simulink model "generic_20231123_1032"  (R2022b)
settings: Solver=ode45  StartTime=0.0  StopTime=50  RelTol=1e-3  EnableMultiTasking=on
model workspace (MAT data in the model file):
  A = 1
  Amplifier = -9.10007585438
  B = 1.19071237887
  K_d_yawrate = 0.231634180251
  K_dsteering = 5.24463953925
  k_speed = -0.570636497542
  k_stanley = 28.4909595466
  kd = -9.99955278144
  ki = 0.00519416981022
  kp = 9.99999979837
  path_curvature = 0
values from neighbouring files (symbols this model uses):
  brake_select = ones(length(speed), length(steering_angle))    [TwoDLook_uptable.m]
  curvature = 0.000:0.001:1    [TwoDLook_uptable.m]
  m = 1600    [MPCController1.m]    (also in MPCController2.m; MPC_Fmincon.m)
  speed = 0:0.1:100    [TwoDLook_uptable.m]
  steering_angle = -3.14/4:0.00628/4:3.14/4    [TwoDLook_uptable.m]
undefined symbols (not defined in the file or in its folder): DiscIntNeverNeededParam
libraries: CarMaker4SL x143, simulink x11, cstblocks x6, simulink_extras x4, autolibshared x1, mpcadaslib x1
(part 3 of 7)

== system generic_20231123_1032/CarMaker/IPG Vehicle/CarAndTrailer/Forces/Vehicle Forces ==
  Sync_In : Inport
  Bus Creator1 : BusCreator  Inputs=12
  Bus Creator8 : BusCreator  Inputs=16
  BusCreator1 : BusCreator  Inputs=4
  BusCreator2 : BusCreator  Inputs=9
  Demux : Demux  Outputs=16
      settings: DisplayOption=none
  Demux1 : Demux  Outputs=12
      settings: DisplayOption=none
  Demux2 : Demux  Outputs=13
      settings: DisplayOption=none
  Forces : S-Function  FunctionName=CM_Sfun  Parameters='Forces'  SFunctionDeploymentMode=off  EnableBusSupport=off
  Terminator : Terminator
  Sync_Out : Outport  VectorParamsAs1DForOutWhenUnconnected=off
  Car.Virtual : Outport  Port=2  VectorParamsAs1DForOutWhenUnconnected=off
  Car.Aero : Outport  Port=3  VectorParamsAs1DForOutWhenUnconnected=off
  Car.Load : Outport  Port=4  VectorParamsAs1DForOutWhenUnconnected=off
  wires:
  BusCreator1/1 -> Terminator/1  "Aero IF (in)"
  Demux2/13 -> BusCreator2/9  "car Aero Trq_1 z"
  Demux2/12 -> BusCreator2/8  "car Aero Trq_1 y"
  Demux2/11 -> BusCreator2/7  "car Aero Trq_1 x"
  Demux2/10 -> BusCreator2/6  "car Aero Frc_1 z"
  Demux2/9 -> BusCreator2/5  "car Aero Frc_1 y"
  Demux2/8 -> BusCreator2/4  "car Aero Frc_1 x"
  Demux2/7 -> BusCreator2/3  "car Aero PoA_1 z"
  Demux2/6 -> BusCreator2/2  "car Aero PoA_1 y"
  Demux2/5 -> BusCreator2/1  "car Aero PoA_1 x"
  Demux2/4 -> BusCreator1/4  "car Aero tau_1"
  Demux2/3 -> BusCreator1/3  "car Aero ApproachVel_1 z"
  Demux2/2 -> BusCreator1/2  "car Aero ApproachVel_1 y"
  Demux2/1 -> BusCreator1/1  "car Aero ApproachVel_1 x"
  Demux/16 -> Bus Creator8/16  "Car Load_3 tz"
  Demux/15 -> Bus Creator8/15  "Car Load_3 ty"
  Demux/14 -> Bus Creator8/14  "Car Load_3 tx"
  Demux/13 -> Bus Creator8/13  "Car Load_3 mass"
  Demux1/12 -> Bus Creator1/12  "Car Virtual Trq_0 z"
  Demux1/11 -> Bus Creator1/11  "Car Virtual Trq_0 y"
  Demux1/10 -> Bus Creator1/10  "Car Virtual Trq_0 x"
  Demux1/9 -> Bus Creator1/9  "Car Virtual Trq_1 z"
  Demux1/8 -> Bus Creator1/8  "Car Virtual Trq_1 y"
  Demux1/7 -> Bus Creator1/7  "Car Virtual Trq_1 x"
  Demux1/6 -> Bus Creator1/6  "Car Virtual Frc_0 z"
  Demux1/5 -> Bus Creator1/5  "Car Virtual Frc_0 y"
  Demux1/4 -> Bus Creator1/4  "Car Virtual Frc_0 x"
  Sync_In/1 -> Forces/1
  Forces/1 -> Sync_Out/1
  BusCreator2/1 -> Car.Aero/1
  Demux1/1 -> Bus Creator1/1  "Car Virtual Frc_1 x"
  Demux1/2 -> Bus Creator1/2  "Car Virtual Frc_1 y"
  Demux1/3 -> Bus Creator1/3  "Car Virtual Frc_1 z"
  Forces/3 -> Demux2/1
  Forces/2 -> Demux1/1
  Bus Creator1/1 -> Car.Virtual/1
  Bus Creator8/1 -> Car.Load/1
  Demux/1 -> Bus Creator8/1  "Car Load_0 mass"
  Demux/2 -> Bus Creator8/2  "Car Load_0 tx"
  Demux/3 -> Bus Creator8/3  "Car Load_0 ty"
  Demux/4 -> Bus Creator8/4  "Car Load_0 tz"
  Demux/5 -> Bus Creator8/5  "Car Load_1 mass"
  Demux/6 -> Bus Creator8/6  "Car Load_1 tx"
  Demux/7 -> Bus Creator8/7  "Car Load_1 ty"
  Demux/8 -> Bus Creator8/8  "Car Load_1 tz"
  Demux/9 -> Bus Creator8/9  "Car Load_2 mass"
  Demux/10 -> Bus Creator8/10  "Car Load_2 tx"
  Demux/11 -> Bus Creator8/11  "Car Load_2 ty"
  Demux/12 -> Bus Creator8/12  "Car Load_2 tz"
  Forces/4 -> Demux/1

== system generic_20231123_1032/CarMaker/IPG Vehicle/CarAndTrailer/Trailer/CreateBus Car.Hitch.FrcTrq ==
  In1 : Inport
  Bus Creator7 : BusCreator  Inputs=6
  Demux7 : Demux  Outputs=6
      settings: DisplayOption=none
  Out1 : Outport  VectorParamsAs1DForOutWhenUnconnected=off
  wires:
  In1/1 -> Demux7/1
  Bus Creator7/1 -> Out1/1
  Demux7/6 -> Bus Creator7/6  "Car Hitch Trq2Car z"
  Demux7/5 -> Bus Creator7/5  "Car Hitch Trq2Car y"
  Demux7/4 -> Bus Creator7/4  "Car Hitch Trq2Car x"
  Demux7/3 -> Bus Creator7/3  "Car Hitch Frc2Car z"
  Demux7/2 -> Bus Creator7/2  "Car Hitch Frc2Car y"
  Demux7/1 -> Bus Creator7/1  "Car Hitch Frc2Car x"

== system generic_20231123_1032/CarMaker/IPG Vehicle/CarAndTrailer/Trailer/CreateBus Vhcl.Motion ==
  In1 : Inport
  BusCreator : BusCreator  Inputs=15
  Demux : Demux  Outputs=15
      settings: DisplayOption=none
  Out1 : Outport  VectorParamsAs1DForOutWhenUnconnected=off
  wires:
  Demux/15 -> BusCreator/15  "Vhcl YawAcc"
  Demux/14 -> BusCreator/14  "Vhcl YawVel"
  Demux/13 -> BusCreator/13  "Vhcl Yaw"
  Demux/12 -> BusCreator/12  "Vhcl PitchAcc"
  Demux/11 -> BusCreator/11  "Vhcl PitchVel"
  Demux/10 -> BusCreator/10  "Vhcl Pitch"
  Demux/9 -> BusCreator/9  "Vhcl RollAcc"
  Demux/8 -> BusCreator/8  "Vhcl RollVel"
  Demux/7 -> BusCreator/7  "Vhcl Roll"
  Demux/6 -> BusCreator/6  "Vhcl Hitch_Pos z"
  Demux/5 -> BusCreator/5  "Vhcl Hitch_Pos y"
  Demux/4 -> BusCreator/4  "Vhcl Hitch_Pos x"
  Demux/3 -> BusCreator/3  "Vhcl sRoad"
  Demux/2 -> BusCreator/2  "Vhcl Distance"
  Demux/1 -> BusCreator/1  "Vhcl v"
  In1/1 -> Demux/1
  BusCreator/1 -> Out1/1

== system generic_20231123_1032/CarMaker/IPG Vehicle/CarAndTrailer/Trailer/CreateBus Vhcl.PoI ==
  In1 : Inport
  Bus Creator3 : BusCreator  Inputs=18
  Demux3 : Demux  Outputs=18
      settings: DisplayOption=none
  Out1 : Outport  VectorParamsAs1DForOutWhenUnconnected=off
  wires:
  Demux3/18 -> Bus Creator3/18  "Vhcl PoI_GCS Elev"
  Demux3/17 -> Bus Creator3/17  "Vhcl PoI_GCS Lat"
  Demux3/16 -> Bus Creator3/16  "Vhcl PoI_GCS Long"
  Demux3/15 -> Bus Creator3/15  "Vhcl PoI_Acc_1 z"
  Demux3/14 -> Bus Creator3/14  "Vhcl PoI_Acc_1 y"
  Demux3/13 -> Bus Creator3/13  "Vhcl PoI_Acc_1 x"
  Demux3/12 -> Bus Creator3/12  "Vhcl PoI_Vel_1 z"
  Demux3/11 -> Bus Creator3/11  "Vhcl PoI_Vel_1 y"
  Demux3/10 -> Bus Creator3/10  "Vhcl PoI_Vel_1 x"
  Demux3/9 -> Bus Creator3/9  "Vhcl PoI_Acc z"
  Demux3/8 -> Bus Creator3/8  "Vhcl PoI_Acc y"
  Demux3/7 -> Bus Creator3/7  "Vhcl PoI_Acc x"
  Demux3/6 -> Bus Creator3/6  "Vhcl PoI_Vel z"
  Demux3/5 -> Bus Creator3/5  "Vhcl PoI_Vel y"
  Demux3/4 -> Bus Creator3/4  "Vhcl PoI_Vel x"
  Demux3/3 -> Bus Creator3/3  "Vhcl PoI_Pos z"
  Demux3/2 -> Bus Creator3/2  "Vhcl PoI_Pos y"
  In1/1 -> Demux3/1
  Bus Creator3/1 -> Out1/1
  Demux3/1 -> Bus Creator3/1  "Vhcl PoI_Pos x"

== system generic_20231123_1032/CarMaker/IPG Vehicle/CarAndTrailer/Trailer/CreateBus Vhcl.Steering ==
  In1 : Inport
  Bus Creator3 : BusCreator  Inputs=4
  Demux : Demux
      settings: DisplayOption=none
  Out1 : Outport  VectorParamsAs1DForOutWhenUnconnected=off
  wires:
  Bus Creator3/1 -> Out1/1
  Demux/1 -> Bus Creator3/1  "Vhcl Steering Ang"
  Demux/3 -> Bus Creator3/3  "Vhcl Steering AngAcc"
  Demux/2 -> Bus Creator3/2  "Vhcl Steering AngVel"
  Demux/4 -> Bus Creator3/4  "Vhcl Steering Trq"
  In1/1 -> Demux/1

== system generic_20231123_1032/CarMaker/IPG Vehicle/CarAndTrailer/Trailer/CreateBus Vhcl.Wheel.FL ==
  In1 : Inport
  Bus Creator3 : BusCreator  Inputs=14
  Demux3 : Demux  Outputs=14
      settings: DisplayOption=none
  Out1 : Outport  VectorParamsAs1DForOutWhenUnconnected=off
  wires:
  Demux3/14 -> Bus Creator3/14  "Vhcl Wheel FL Trq_WhlBearing"
  Demux3/13 -> Bus Creator3/13  "Vhcl Wheel FL Trq_T2W"
  Demux3/12 -> Bus Creator3/12  "Vhcl Wheel FL SideSlip"
  Demux3/11 -> Bus Creator3/11  "Vhcl Wheel FL LongSlip"
  Demux3/10 -> Bus Creator3/10  "Vhcl Wheel FL vBelt"
  Demux3/9 -> Bus Creator3/9  "Vhcl Wheel FL Fz"
  Demux3/8 -> Bus Creator3/8  "Vhcl Wheel FL Fy"
  Demux3/7 -> Bus Creator3/7  "Vhcl Wheel FL Fx"
  Demux3/6 -> Bus Creator3/6  "Vhcl Wheel FL r_zxy z"
  Demux3/5 -> Bus Creator3/5  "Vhcl Wheel FL r_zxy y"
  Demux3/4 -> Bus Creator3/4  "Vhcl Wheel FL r_zxy x"
  Demux3/3 -> Bus Creator3/3  "Vhcl Wheel FL t z"
  Demux3/2 -> Bus Creator3/2  "Vhcl Wheel FL t y"
  In1/1 -> Demux3/1
  Bus Creator3/1 -> Out1/1
  Demux3/1 -> Bus Creator3/1  "Vhcl Wheel FL t x"

== system generic_20231123_1032/CarMaker/IPG Vehicle/CarAndTrailer/Trailer/CreateBus Vhcl.Wheel.FR ==
  In1 : Inport
  Bus Creator3 : BusCreator  Inputs=14
  Demux3 : Demux  Outputs=14
      settings: DisplayOption=none
  Out1 : Outport  VectorParamsAs1DForOutWhenUnconnected=off
  wires:
  Demux3/14 -> Bus Creator3/14  "Vhcl Wheel FR Trq_WhlBearing"
  Demux3/13 -> Bus Creator3/13  "Vhcl Wheel FR Trq_T2W"
  Demux3/12 -> Bus Creator3/12  "Vhcl Wheel FR SideSlip"
  Demux3/11 -> Bus Creator3/11  "Vhcl Wheel FR LongSlip"
  Demux3/10 -> Bus Creator3/10  "Vhcl Wheel FR vBelt"
  Demux3/9 -> Bus Creator3/9  "Vhcl Wheel FR Fz"
  Demux3/8 -> Bus Creator3/8  "Vhcl Wheel FR Fy"
  Demux3/7 -> Bus Creator3/7  "Vhcl Wheel FR Fx"
  Demux3/6 -> Bus Creator3/6  "Vhcl Wheel FR r_zxy z"
  Demux3/5 -> Bus Creator3/5  "Vhcl Wheel FR r_zxy y"
  Demux3/4 -> Bus Creator3/4  "Vhcl Wheel FR r_zxy x"
  Demux3/3 -> Bus Creator3/3  "Vhcl Wheel FR t z"
  Demux3/2 -> Bus Creator3/2  "Vhcl Wheel FR t y"
  In1/1 -> Demux3/1
  Bus Creator3/1 -> Out1/1
  Demux3/1 -> Bus Creator3/1  "Vhcl Wheel FR t x"

== system generic_20231123_1032/CarMaker/IPG Vehicle/CarAndTrailer/Trailer/CreateBus Vhcl.Wheel.RL ==
  In1 : Inport
  Bus Creator3 : BusCreator  Inputs=14
  Demux3 : Demux  Outputs=14
      settings: DisplayOption=none
  Out1 : Outport  VectorParamsAs1DForOutWhenUnconnected=off
  wires:
  Demux3/14 -> Bus Creator3/14  "Vhcl Wheel RL Trq_WhlBearing"
  Demux3/13 -> Bus Creator3/13  "Vhcl Wheel RL Trq_T2W"
  Demux3/12 -> Bus Creator3/12  "Vhcl Wheel RL SideSlip"
  Demux3/11 -> Bus Creator3/11  "Vhcl Wheel RL LongSlip"
  Demux3/10 -> Bus Creator3/10  "Vhcl Wheel RL vBelt"
  Demux3/9 -> Bus Creator3/9  "Vhcl Wheel RL Fz"
  Demux3/8 -> Bus Creator3/8  "Vhcl Wheel RL Fy"
  Demux3/7 -> Bus Creator3/7  "Vhcl Wheel RL Fx"
  Demux3/6 -> Bus Creator3/6  "Vhcl Wheel RL r_zxy z"
  Demux3/5 -> Bus Creator3/5  "Vhcl Wheel RL r_zxy y"
  Demux3/4 -> Bus Creator3/4  "Vhcl Wheel RL r_zxy x"
  Demux3/3 -> Bus Creator3/3  "Vhcl Wheel RL t z"
  Demux3/2 -> Bus Creator3/2  "Vhcl Wheel RL t y"
  In1/1 -> Demux3/1
  Bus Creator3/1 -> Out1/1
  Demux3/1 -> Bus Creator3/1  "Vhcl Wheel RL t x"

== system generic_20231123_1032/CarMaker/IPG Vehicle/CarAndTrailer/Trailer/CreateBus Vhcl.Wheel.RR ==
  In1 : Inport
  Bus Creator3 : BusCreator  Inputs=14
  Demux3 : Demux  Outputs=14
      settings: DisplayOption=none
  Out1 : Outport  VectorParamsAs1DForOutWhenUnconnected=off
  wires:
  Demux3/14 -> Bus Creator3/14  "Vhcl Wheel RR Trq_WhlBearing"
  Demux3/13 -> Bus Creator3/13  "Vhcl Wheel RR Trq_T2W"
  Demux3/12 -> Bus Creator3/12  "Vhcl Wheel RR SideSlip"
  Demux3/11 -> Bus Creator3/11  "Vhcl Wheel RR LongSlip"
  Demux3/10 -> Bus Creator3/10  "Vhcl Wheel RR vBelt"
  Demux3/9 -> Bus Creator3/9  "Vhcl Wheel RR Fz"
  Demux3/8 -> Bus Creator3/8  "Vhcl Wheel RR Fy"
  Demux3/7 -> Bus Creator3/7  "Vhcl Wheel RR Fx"
  Demux3/6 -> Bus Creator3/6  "Vhcl Wheel RR r_zxy z"
  Demux3/5 -> Bus Creator3/5  "Vhcl Wheel RR r_zxy y"
  Demux3/4 -> Bus Creator3/4  "Vhcl Wheel RR r_zxy x"
  Demux3/3 -> Bus Creator3/3  "Vhcl Wheel RR t z"
  Demux3/2 -> Bus Creator3/2  "Vhcl Wheel RR t y"
  In1/1 -> Demux3/1
  Bus Creator3/1 -> Out1/1
  Demux3/1 -> Bus Creator3/1  "Vhcl Wheel RR t x"

== system generic_20231123_1032/CarMaker/VehicleControl/CreateBus VhclCtrl/A*algoithm/Subsystem ==
  Bus Selector : BusSelector  OutputSignals=Route.tx,Route.ty
  Constant : Constant  Value=0
  Constant1 : Constant  Value=0
  Read CM Dict : CarMaker4SL/Read CM Dict  xname=Sensor.Radar.VehSensor_6.Obj0.DistX  xsync=off  xstime=Continuous
  Read CM Dict1 : CarMaker4SL/Read CM Dict  xname=Sensor.Radar.VehSensor_6.Obj0.DistY  xsync=off  xstime=Continuous
  Read CM Dict3 : CarMaker4SL/Read CM Dict  xname=Sensor.Radar.VehSensor_6.Obj0.ProbObst  xsync=off  xstime=Continuous
  Road Sensor : CarMaker4SL/Sensors/Road Sensor  xname=0  xstime=Continuous
      settings: SourceProductName=CarMaker4SL
  Sum : Sum  Inputs=|++
  Sum1 : Sum  Inputs=|++
  Switch : Switch  Criteria=u2 > Threshold  SaturateOnIntegerOverflow=off  InputSameDT=off
  Switch1 : Switch  Criteria=u2 > Threshold  SaturateOnIntegerOverflow=off  InputSameDT=off
  Out1 : Outport
  Out2 : Outport  Port=2
  Out3 : Outport  Port=3
  wires:
  Read CM Dict1/1 -> Sum/1
  Sum/1 -> Switch/1
  Constant/1 -> Switch1/3, Switch/3
  Sum1/1 -> Switch1/1
  Switch/1 -> Out1/1
  Bus Selector/2 -> Sum1/1  "<ty>"
  Read CM Dict3/1 -> Switch1/2, Switch/2
  Read CM Dict/1 -> Sum1/2
  Road Sensor/2 -> Bus Selector/1
  Constant1/1 -> Road Sensor/1
  Bus Selector/1 -> Sum/2  "<tx>"
  Road Sensor/1 -> Out3/1
  Switch1/1 -> Out2/1

== system generic_20231123_1032/CarMaker/VehicleControl/CreateBus VhclCtrl/MPC_steering_controllers/State_space_system_variables ==
  Yaw_ref_deg : Inport
  Y_ref_m : Inport  Port=2
  X_ref_m : Inport  Port=3
  Discrete-Time Integrator2 : DiscreteIntegrator  SampleTime=-1  ICPrevOutput=DiscIntNeverNeededParam  ICPrevScaledInput=DiscIntNeverNeededParam
  Gain : Gain  Gain=3.6
  Mux : Mux  Inputs=8
  Radians to Degrees2 : simulink_extras/Transformations/Radians to Degrees
  Radians to Degrees3 : simulink_extras/Transformations/Radians to Degrees
  Read CM Dict10 : CarMaker4SL/Read CM Dict  xname=Car.Gen.tx  xsync=off  xstime=Continuous
  Read CM Dict2 : CarMaker4SL/Read CM Dict  xname=Car.YawRate  xsync=off  xstime=Continuous
  Read CM Dict3 : CarMaker4SL/Read CM Dict  xname=Car.YawRate  xsync=off  xstime=Continuous
  Read CM Dict4 : CarMaker4SL/Read CM Dict  xname=Car.Gen.tx  xsync=off  xstime=Continuous
  Read CM Dict5 : CarMaker4SL/Read CM Dict  xname=Car.Gen.ty  xsync=off  xstime=Continuous
  Read CM Dict6 : CarMaker4SL/Read CM Dict  xname=Car.Con.vy_1  xsync=off  xstime=Continuous
  Read CM Dict7 : CarMaker4SL/Read CM Dict  xname=Car.Con.vx_1  xsync=off  xstime=Continuous
  Scope : Scope
  Sum : Sum  Inputs=|++
  Terminator : Terminator
  Terminator1 : Terminator
  Vlocity_correction : Constant
  x : Outport
  Lateral_velocity : Outport  Port=2
  wires:
  Vlocity_correction/1 -> Sum/2
  Read CM Dict4/1 -> Terminator/1
  Read CM Dict2/1 -> Discrete-Time Integrator2/1
  Radians to Degrees3/1 -> Mux/2
  Discrete-Time Integrator2/1 -> Scope/1, Radians to Degrees3/1
  Read CM Dict6/1 -> Gain/1
  Read CM Dict3/1 -> Radians to Degrees2/1
  Read CM Dict7/1 -> Sum/1  "Longitudinal_velocity"
  Gain/1 -> Mux/1, Lateral_velocity/1
  Radians to Degrees2/1 -> Mux/3
  Read CM Dict5/1 -> Mux/4
  Read CM Dict10/1 -> Mux/5
  Y_ref_m/1 -> Terminator1/1
  Yaw_ref_deg/1 -> Mux/7
  Sum/1 -> Mux/8
  Mux/1 -> x/1  "x"
  X_ref_m/1 -> Mux/6

== system generic_20231123_1032/CarMaker/VehicleControl/CreateBus VhclCtrl/MPC_steering_controllers/Subsystem ==
  x : Inport
  u : Inport  Port=2
  dt : Inport  Port=3
  dev : Inport  Port=4
  Constant4 : Constant  Commented=on  Value=B
  Constant5 : Constant  Value=21543*180/pi()
  Constant6 : Constant  Value=70551*180/pi()
  MATLAB Function1 : MATLAB Function  Commented=on  TreatAsAtomicUnit=on
  MATLAB Function2 : MATLAB Function  Commented=on  TreatAsAtomicUnit=on
  MATLAB Function3 : MATLAB Function  Commented=on  TreatAsAtomicUnit=on
  MATLAB Function4 : MATLAB Function  Commented=on  TreatAsAtomicUnit=on
  MATLAB Function5 : MATLAB Function  Commented=on  TreatAsAtomicUnit=on
  MATLAB Function6 : MATLAB Function  Commented=on  TreatAsAtomicUnit=on
  MATLAB Function7 : MATLAB Function  Commented=on  TreatAsAtomicUnit=on
  S-Function : S-Function  Commented=on  FunctionName=MPCController2  SFunctionDeploymentMode=off  EnableBusSupport=off
  u_optimal : Outport
  steering : Outport  Port=2
  x_new : Outport  Port=3
  theta_new : Outport  Port=4
  wires:
  Constant4/1 -> MATLAB Function1/2(B)
  dt/1 -> MATLAB Function3/3(dt)
  u/1 -> MATLAB Function3/2(u)
  x/1 -> MATLAB Function3/1(x)
  MATLAB Function3/1(u_optimal) -> u_optimal/1
  MATLAB Function3/3(theta_new) -> theta_new/1
  MATLAB Function1/1(steering) -> steering/1
  MATLAB Function3/2(x_new) -> x_new/1
  dev/1 -> MATLAB Function1/1(dev)
  MATLAB Function2/1(delta) -> ?

== system generic_20231123_1032/CarMaker/VehicleControl/CreateBus VhclCtrl/MPC_steering_controllers/Traditional_MPC ==
  Lateral_deviation : Inport
  Dev_angle : Inport  Port=2
  Constant8 : Constant  Value=A
  Constant9 : Constant  Value=B
  MPC_steering_control : MATLAB Function  TreatAsAtomicUnit=on
  MPC_steering_control1 : MATLAB Function  TreatAsAtomicUnit=on
  Sum1 : Sum  Inputs=|++
  steering_cmd : Outport
  Heading_correction : Outport  Port=2
  wires:
  Dev_angle/1 -> MPC_steering_control1/1(Heading_error)
  Lateral_deviation/1 -> MPC_steering_control/1(Lateral_deviation)
  Constant9/1 -> MPC_steering_control/3(B), MPC_steering_control1/3(B)
  Constant8/1 -> MPC_steering_control1/2(A), MPC_steering_control/2(A)
  MPC_steering_control/1(steering_cmd) -> Sum1/1
  MPC_steering_control1/1(steering_cmd) -> Heading_correction/1, Sum1/2
  Sum1/1 -> steering_cmd/1

== system generic_20231123_1032/CarMaker/VehicleControl/CreateBus VhclCtrl/PID steering controller/Dervative ==
  Error : Inport
  Discrete Derivative : simulink/Discrete/Discrete Derivative  gainval=1.0  ICPrevScaledInput=0.01  OutMin=[]  OutMax=[]  OutDataType=fixdt(1, 16)  OutScaling=2^-10  DoSatur=off
  Gain2 : Gain  Gain=0.4
  Dervative term : Outport
  wires:
  Error/1 -> Gain2/1
  Gain2/1 -> Discrete Derivative/1
  Discrete Derivative/1 -> Dervative term/1

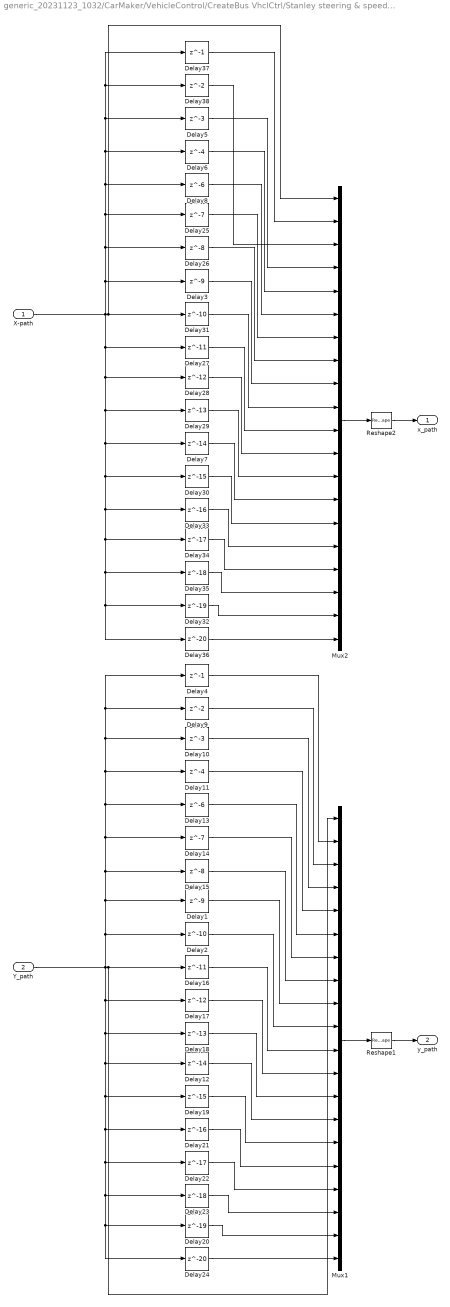
== system generic_20231123_1032/CarMaker/VehicleControl/CreateBus VhclCtrl/Stanley steering & speed//Brake controller/ Path_expanding ==
  X-path : Inport
  Y_path : Inport  Port=2
  Delay1 : Delay  DelayLength=9
  Delay10 : Delay  DelayLength=3
  Delay11 : Delay  DelayLength=4
  Delay12 : Delay  DelayLength=14
  Delay13 : Delay  DelayLength=6
  Delay14 : Delay  DelayLength=7
  Delay15 : Delay  DelayLength=8
  Delay16 : Delay  DelayLength=11
  Delay17 : Delay  DelayLength=12
  Delay18 : Delay  DelayLength=13
  Delay19 : Delay  DelayLength=15
  Delay2 : Delay  DelayLength=10
  Delay20 : Delay  DelayLength=19
  Delay21 : Delay  DelayLength=16
  Delay22 : Delay  DelayLength=17
  Delay23 : Delay  DelayLength=18
  Delay24 : Delay  DelayLength=20
  Delay25 : Delay  DelayLength=7
  Delay26 : Delay  DelayLength=8
  Delay27 : Delay  DelayLength=11
  Delay28 : Delay  DelayLength=12
  Delay29 : Delay  DelayLength=13
  Delay3 : Delay  DelayLength=9
  Delay30 : Delay  DelayLength=15
  Delay31 : Delay  DelayLength=10
  Delay32 : Delay  DelayLength=19
  Delay33 : Delay  DelayLength=16
  Delay34 : Delay  DelayLength=17
  Delay35 : Delay  DelayLength=18
  Delay36 : Delay  DelayLength=20
  Delay37 : Delay  DelayLength=1
  Delay38 : Delay
  Delay4 : Delay  DelayLength=1
  Delay5 : Delay  DelayLength=3
  Delay6 : Delay  DelayLength=4
  Delay7 : Delay  DelayLength=14
  Delay8 : Delay  DelayLength=6
  Delay9 : Delay
  Mux1 : Mux  Inputs=20
  Mux2 : Mux  Inputs=20
  Reshape1 : Reshape  OutputDimensionality=Customize  OutputDimensions=[1,20]
  Reshape2 : Reshape  OutputDimensionality=Customize  OutputDimensions=[1,20]
  x_path : Outport
  y_path : Outport  Port=2
  wires:
  Delay12/1 -> Mux1/14
  X-path/1 -> Delay32/1, Delay36/1, Delay35/1, Delay34/1, Delay33/1, Delay30/1, Delay7/1, Delay29/1, Delay28/1, Delay27/1, Delay31/1, Mux2/1, Delay38/1, Delay37/1, Delay5/1, Delay6/1, Delay8/1, Delay25/1, Delay26/1, Delay3/1
  Delay25/1 -> Mux2/7
  Delay17/1 -> Mux1/12
  Y_path/1 -> Delay20/1, Delay24/1, Delay23/1, Delay22/1, Delay21/1, Delay19/1, Delay12/1, Delay18/1, Delay17/1, Mux1/1, Delay16/1, Delay4/1, Delay9/1, Delay10/1, Delay11/1, Delay13/1, Delay14/1, Delay15/1, Delay1/1, Delay2/1
  Delay5/1 -> Mux2/4
  Delay37/1 -> Mux2/2
  Delay6/1 -> Mux2/5
  Delay38/1 -> Mux2/3
  Delay20/1 -> Mux1/19
  Delay18/1 -> Mux1/13
  Delay8/1 -> Mux2/6
  Delay26/1 -> Mux2/8
  Delay3/1 -> Mux2/9
  Delay31/1 -> Mux2/10
  Delay27/1 -> Mux2/11
  Delay24/1 -> Mux1/20
  Delay28/1 -> Mux2/12
  Delay29/1 -> Mux2/13
  Delay7/1 -> Mux2/14
  Delay30/1 -> Mux2/15
  Delay33/1 -> Mux2/16
  Mux1/1 -> Reshape1/1
  Delay34/1 -> Mux2/17
  Delay35/1 -> Mux2/18
  Delay1/1 -> Mux1/9
  Delay32/1 -> Mux2/19
  Delay15/1 -> Mux1/8
  Delay36/1 -> Mux2/20
  Reshape1/1 -> y_path/1
  Delay4/1 -> Mux1/2
  Delay16/1 -> Mux1/11
  Delay9/1 -> Mux1/3
  Delay21/1 -> Mux1/16
  Delay10/1 -> Mux1/4
  Delay11/1 -> Mux1/5
  Delay13/1 -> Mux1/6
  Reshape2/1 -> x_path/1
  Delay14/1 -> Mux1/7
  Delay2/1 -> Mux1/10
  Delay19/1 -> Mux1/15
  Delay22/1 -> Mux1/17
  Delay23/1 -> Mux1/18
  Mux2/1 -> Reshape2/1

== system generic_20231123_1032/CarMaker/VehicleControl/CreateBus VhclCtrl/Stanley steering & speed//Brake controller/Road sensor set & path planning ==
  Road sensor set & path planning : Subsystem  VariantControl=Choice
  <tx> : Outport
  <ty> : Outport  Port=2
  <DevDist> : Outport  Port=3
  <CurveXY> : Outport  Port=4
  Yaw_rate : Outport  Port=5
  Velocity_m_s : Outport  Port=6
  smoothed_path_curvature : Outport  Port=7

== system generic_20231123_1032/CarMaker/VehicleControl/CreateBus VhclCtrl/Stanley steering & speed//Brake controller/Stanley controller version_1 ==
  Direction : Inport
  Stanley controller version_1 : Subsystem  VariantControl=Choice  ReferencedSubsystem=Stanley_controller_version_1
  Radians out : Outport
  SteerCmd : Outport  Port=2

== system generic_20231123_1032/CarMaker/VehicleControl/CreateBus VhclCtrl/Stanley steering & speed//Brake controller/Stanley controller with path_planning ==
  X-path : Inport
  Y_path : Inport  Port=2
  Stanley controller with path_planning : Subsystem  VariantControl=Choice
  e : Outport
  err_fr_axle : Outport  Port=2
  cross_track_steering : Outport  Port=3
  heading_err : Outport  Port=4
  Steering : Outport  Port=5
  closest_point : Outport  Port=6

== system generic_20231123_1032/CarMaker/VehicleControl/CreateBus VhclCtrl/Stanley steering & speed//Brake controller/Stanley_controller_vfin ==
  Velocity : Inport
  Curvature : Inport  Port=2
  Vehicle_yaw_rate : Inport  Port=3
  Path.DevDist : Inport  Port=4
  Stanley_controller_vfin : Subsystem  Variant=on  VariantControlMode=label  VariantControl=Choice  LabelModeActiveChoice=Choice
  Steering angle : Outport
  dev_angle : Outport  Port=2

== system generic_20231123_1032/CarMaker/VehicleControl/CreateBus VhclCtrl/Stanley steering & speed//Brake controller/Stanley_controller_with_thottle_and_brake_commands ==
  Path Out : Inport
  dev_angle : Inport  Port=2
  dev_distance : Inport  Port=3
  smoothed_path_curvature : Inport  Port=4
  Desired_speed : Inport  Port=5
  Abs : Abs  SaturateOnIntegerOverflow=off
  Abs1 : Abs  SaturateOnIntegerOverflow=off
  Constant : Constant
  Constant1 : Constant
  Constant5 : Constant  Value=2
  MPCLongitudianl_contorl : Subsystem
  Memory3 : Memory
  Memory4 : Memory
  Stanley steering + PID speed controller : Subsystem
  Terminator : Terminator
  Throttle_selector : MultiPortSwitch  Inputs=2  SaturateOnIntegerOverflow=off  InputSameDT=off
  Target_Steering_angle_rad : Outport
  Throttle : Outport  Port=2
  Brake_command : Outport  Port=3
  wires:
  dev_angle/1 -> [dev_angle]
  Memory4/1 -> Stanley steering + PID speed controller/2(<Vx_Global_m_s>)
  Constant/1 -> Abs/1
  [dev_angle] -> Stanley steering + PID speed controller/4(dev_angle)
  smoothed_path_curvature/1 -> MPCLongitudianl_contorl/1(smoothed_path_curvature)
  Stanley steering + PID speed controller/1(Steering_angle_rad) -> MPCLongitudianl_contorl/3(steering_angle), Target_Steering_angle_rad/1
  Constant1/1 -> Abs1/1
  Path Out/1 -> Stanley steering + PID speed controller/1(Path_out)
  Abs/1 -> Memory4/1
  Constant5/1 -> Throttle_selector/1
  Abs1/1 -> Memory3/1
  Memory3/1 -> Stanley steering + PID speed controller/3(<Vy_Global_m_s>)
  MPCLongitudianl_contorl/1(actual_velocity) -> Stanley steering + PID speed controller/5(<Actual_Velocity_Car_m_s>)  "actual_velocity"
  MPCLongitudianl_contorl/3(throttle) -> Throttle_selector/3  "throttle"
  MPCLongitudianl_contorl/2(Deisred_speed) -> Stanley steering + PID speed controller/6(Desired_speed)  "Deisred_speed"
  dev_distance/1 -> Stanley steering + PID speed controller/7(dev_distance)  "Dev_dis"
  Stanley steering + PID speed controller/3(Brake_command) -> Terminator/1
  Throttle_selector/1 -> Throttle/1
  Desired_speed/1 -> MPCLongitudianl_contorl/2(Desired_speed)
  MPCLongitudianl_contorl/4(Brake) -> Brake_command/1  "Brake_command"
  Stanley steering + PID speed controller/2(Throttle) -> Throttle_selector/2

== system generic_20231123_1032/CarMaker/VehicleControl/CreateBus VhclCtrl/Stanley steering & speed//Brake controller/calculate_path_curvature ==
  path_x : Inport
  path_y : Inport  Port=2
  calculate_path_curvature : ModelReference  ModelNameDialog=calculate_path_curvature  SimulationMode=Normal  VariantControl=Choice  ModelReferenceVersion=6.16
  path_curvature : Outport

== system generic_20231123_1032/CarMaker/VehicleControl/CreateBus VhclCtrl/path_planner_MATLAB/X_Global_Pos_m ==
  In1 : Inport
  Pos_X : Outport  VectorParamsAs1DForOutWhenUnconnected=off
  wires:
  In1/1 -> Pos_X/1

== system generic_20231123_1032/CarMaker/VehicleControl/CreateBus VhclCtrl/path_planner_MATLAB/Y_Global_Pos_m ==
  In1 : Inport
  Pos_Y : Outport  VectorParamsAs1DForOutWhenUnconnected=off
  wires:
  In1/1 -> Pos_Y/1

== system generic_20231123_1032/CarMaker/VehicleControl/CreateBus VhclCtrl/path_planner_MATLAB/Yaw_angle_rad ==
  In1 : Inport
  Yaw_Angle : Outport  VectorParamsAs1DForOutWhenUnconnected=off
  wires:
  In1/1 -> Yaw_Angle/1

== system generic_20231123_1032/CarMaker/VehicleControl/Subsystem1/Obstacle_data_gathering/Subsystem ==
  In1 : Inport
  Add : Sum  Inputs=+++
  Derivative : Derivative
  Discrete-Time Integrator : DiscreteIntegrator  SampleTime=-1  ICPrevOutput=DiscIntNeverNeededParam  ICPrevScaledInput=DiscIntNeverNeededParam
  Gain : Gain  Gain=0.6
  Gain1 : Gain  Gain=1.2
  Gain2 : Gain  Gain=0.4
  Signal_In : Outport
  wires:
  Gain1/1 -> Discrete-Time Integrator/1
  Gain2/1 -> Derivative/1
  Discrete-Time Integrator/1 -> Add/1
  Derivative/1 -> Add/3
  Gain/1 -> Add/2
  In1/1 -> Gain/1, Gain2/1, Gain1/1
  Add/1 -> Signal_In/1

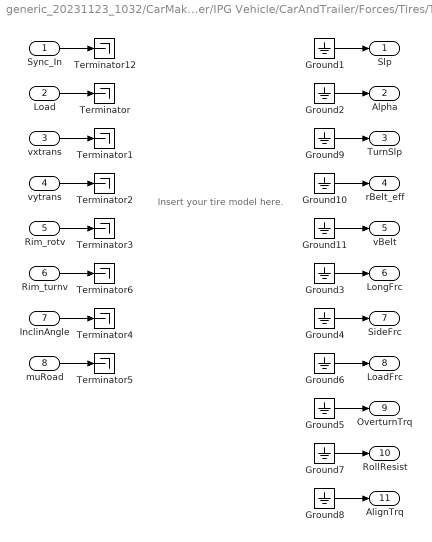
== system generic_20231123_1032/CarMaker/IPG Vehicle/CarAndTrailer/Forces/Tires/TireFL ==
  note: Insert your tire model here.
  Sync_In : Inport
  Load : Inport  Port=2
  vxtrans : Inport  Port=3
  vytrans : Inport  Port=4
  Rim_rotv : Inport  Port=5
  Rim_turnv : Inport  Port=6
  InclinAngle : Inport  Port=7
  muRoad : Inport  Port=8
  Ground{1..11} (11 alike) : Ground
  Terminator{,1..6,12} (8 alike) : Terminator
  Slp : Outport  VectorParamsAs1DForOutWhenUnconnected=off
  Alpha : Outport  Port=2  VectorParamsAs1DForOutWhenUnconnected=off
  TurnSlp : Outport  Port=3  VectorParamsAs1DForOutWhenUnconnected=off
  rBelt_eff : Outport  Port=4  VectorParamsAs1DForOutWhenUnconnected=off
  vBelt : Outport  Port=5  VectorParamsAs1DForOutWhenUnconnected=off
  LongFrc : Outport  Port=6  VectorParamsAs1DForOutWhenUnconnected=off
  SideFrc : Outport  Port=7  VectorParamsAs1DForOutWhenUnconnected=off
  LoadFrc : Outport  Port=8  VectorParamsAs1DForOutWhenUnconnected=off
  OverturnTrq : Outport  Port=9  VectorParamsAs1DForOutWhenUnconnected=off
  RollResist : Outport  Port=10  VectorParamsAs1DForOutWhenUnconnected=off
  AlignTrq : Outport  Port=11  VectorParamsAs1DForOutWhenUnconnected=off
  wires:
  Ground11/1 -> vBelt/1
  Ground10/1 -> rBelt_eff/1
  Ground9/1 -> TurnSlp/1
  Rim_turnv/1 -> Terminator6/1
  Sync_In/1 -> Terminator12/1
  Ground2/1 -> Alpha/1
  Ground3/1 -> LongFrc/1
  Ground4/1 -> SideFrc/1
  Ground5/1 -> OverturnTrq/1
  vxtrans/1 -> Terminator1/1
  vytrans/1 -> Terminator2/1
  Rim_rotv/1 -> Terminator3/1
  InclinAngle/1 -> Terminator4/1
  muRoad/1 -> Terminator5/1
  Load/1 -> Terminator/1
  Ground1/1 -> Slp/1
  Ground6/1 -> LoadFrc/1
  Ground7/1 -> RollResist/1
  Ground8/1 -> AlignTrq/1

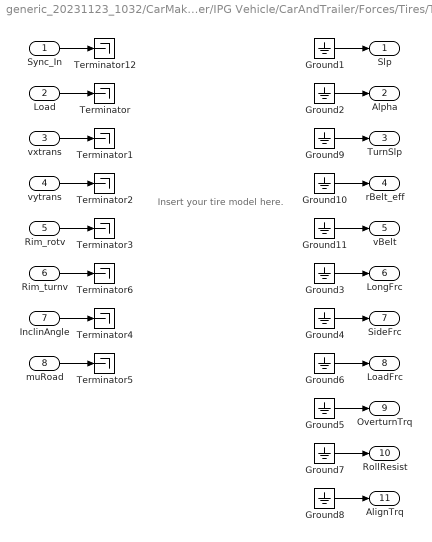
== system generic_20231123_1032/CarMaker/IPG Vehicle/CarAndTrailer/Forces/Tires/TireFR ==
  note: Insert your tire model here.
  Sync_In : Inport
  Load : Inport  Port=2
  vxtrans : Inport  Port=3
  vytrans : Inport  Port=4
  Rim_rotv : Inport  Port=5
  Rim_turnv : Inport  Port=6
  InclinAngle : Inport  Port=7
  muRoad : Inport  Port=8
  Ground{1..11} (11 alike) : Ground
  Terminator{,1..6,12} (8 alike) : Terminator
  Slp : Outport  VectorParamsAs1DForOutWhenUnconnected=off
  Alpha : Outport  Port=2  VectorParamsAs1DForOutWhenUnconnected=off
  TurnSlp : Outport  Port=3  VectorParamsAs1DForOutWhenUnconnected=off
  rBelt_eff : Outport  Port=4  VectorParamsAs1DForOutWhenUnconnected=off
  vBelt : Outport  Port=5  VectorParamsAs1DForOutWhenUnconnected=off
  LongFrc : Outport  Port=6  VectorParamsAs1DForOutWhenUnconnected=off
  SideFrc : Outport  Port=7  VectorParamsAs1DForOutWhenUnconnected=off
  LoadFrc : Outport  Port=8  VectorParamsAs1DForOutWhenUnconnected=off
  OverturnTrq : Outport  Port=9  VectorParamsAs1DForOutWhenUnconnected=off
  RollResist : Outport  Port=10  VectorParamsAs1DForOutWhenUnconnected=off
  AlignTrq : Outport  Port=11  VectorParamsAs1DForOutWhenUnconnected=off
  wires:
  Ground11/1 -> vBelt/1
  Ground10/1 -> rBelt_eff/1
  Ground9/1 -> TurnSlp/1
  Rim_turnv/1 -> Terminator6/1
  Sync_In/1 -> Terminator12/1
  Ground2/1 -> Alpha/1
  Ground3/1 -> LongFrc/1
  Ground4/1 -> SideFrc/1
  Ground5/1 -> OverturnTrq/1
  vxtrans/1 -> Terminator1/1
  vytrans/1 -> Terminator2/1
  Rim_rotv/1 -> Terminator3/1
  InclinAngle/1 -> Terminator4/1
  muRoad/1 -> Terminator5/1
  Load/1 -> Terminator/1
  Ground1/1 -> Slp/1
  Ground6/1 -> LoadFrc/1
  Ground7/1 -> RollResist/1
  Ground8/1 -> AlignTrq/1

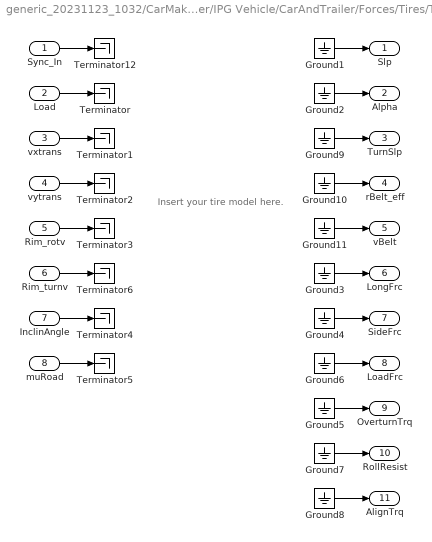
== system generic_20231123_1032/CarMaker/IPG Vehicle/CarAndTrailer/Forces/Tires/TireRL ==
  note: Insert your tire model here.
  Sync_In : Inport
  Load : Inport  Port=2
  vxtrans : Inport  Port=3
  vytrans : Inport  Port=4
  Rim_rotv : Inport  Port=5
  Rim_turnv : Inport  Port=6
  InclinAngle : Inport  Port=7
  muRoad : Inport  Port=8
  Ground{1..11} (11 alike) : Ground
  Terminator{,1..6,12} (8 alike) : Terminator
  Slp : Outport  VectorParamsAs1DForOutWhenUnconnected=off
  Alpha : Outport  Port=2  VectorParamsAs1DForOutWhenUnconnected=off
  TurnSlp : Outport  Port=3  VectorParamsAs1DForOutWhenUnconnected=off
  rBelt_eff : Outport  Port=4  VectorParamsAs1DForOutWhenUnconnected=off
  vBelt : Outport  Port=5  VectorParamsAs1DForOutWhenUnconnected=off
  LongFrc : Outport  Port=6  VectorParamsAs1DForOutWhenUnconnected=off
  SideFrc : Outport  Port=7  VectorParamsAs1DForOutWhenUnconnected=off
  LoadFrc : Outport  Port=8  VectorParamsAs1DForOutWhenUnconnected=off
  OverturnTrq : Outport  Port=9  VectorParamsAs1DForOutWhenUnconnected=off
  RollResist : Outport  Port=10  VectorParamsAs1DForOutWhenUnconnected=off
  AlignTrq : Outport  Port=11  VectorParamsAs1DForOutWhenUnconnected=off
  wires:
  Ground11/1 -> vBelt/1
  Ground10/1 -> rBelt_eff/1
  Ground9/1 -> TurnSlp/1
  Rim_turnv/1 -> Terminator6/1
  Sync_In/1 -> Terminator12/1
  Ground2/1 -> Alpha/1
  Ground3/1 -> LongFrc/1
  Ground4/1 -> SideFrc/1
  Ground5/1 -> OverturnTrq/1
  vxtrans/1 -> Terminator1/1
  vytrans/1 -> Terminator2/1
  Rim_rotv/1 -> Terminator3/1
  InclinAngle/1 -> Terminator4/1
  muRoad/1 -> Terminator5/1
  Load/1 -> Terminator/1
  Ground1/1 -> Slp/1
  Ground6/1 -> LoadFrc/1
  Ground7/1 -> RollResist/1
  Ground8/1 -> AlignTrq/1

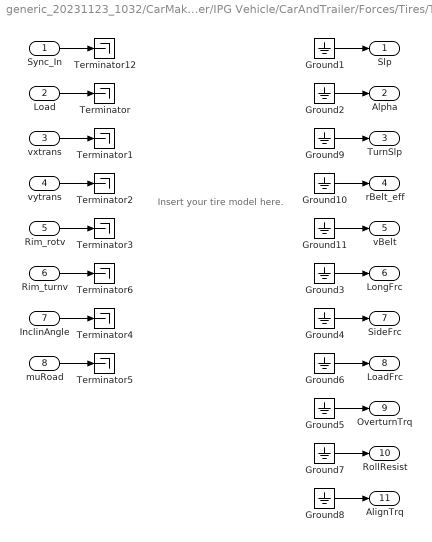
== system generic_20231123_1032/CarMaker/IPG Vehicle/CarAndTrailer/Forces/Tires/TireRR ==
  note: Insert your tire model here.
  Sync_In : Inport
  Load : Inport  Port=2
  vxtrans : Inport  Port=3
  vytrans : Inport  Port=4
  Rim_rotv : Inport  Port=5
  Rim_turnv : Inport  Port=6
  InclinAngle : Inport  Port=7
  muRoad : Inport  Port=8
  Ground{1..11} (11 alike) : Ground
  Terminator{,1..6,12} (8 alike) : Terminator
  Slp : Outport  VectorParamsAs1DForOutWhenUnconnected=off
  Alpha : Outport  Port=2  VectorParamsAs1DForOutWhenUnconnected=off
  TurnSlp : Outport  Port=3  VectorParamsAs1DForOutWhenUnconnected=off
  rBelt_eff : Outport  Port=4  VectorParamsAs1DForOutWhenUnconnected=off
  vBelt : Outport  Port=5  VectorParamsAs1DForOutWhenUnconnected=off
  LongFrc : Outport  Port=6  VectorParamsAs1DForOutWhenUnconnected=off
  SideFrc : Outport  Port=7  VectorParamsAs1DForOutWhenUnconnected=off
  LoadFrc : Outport  Port=8  VectorParamsAs1DForOutWhenUnconnected=off
  OverturnTrq : Outport  Port=9  VectorParamsAs1DForOutWhenUnconnected=off
  RollResist : Outport  Port=10  VectorParamsAs1DForOutWhenUnconnected=off
  AlignTrq : Outport  Port=11  VectorParamsAs1DForOutWhenUnconnected=off
  wires:
  Ground11/1 -> vBelt/1
  Ground10/1 -> rBelt_eff/1
  Ground9/1 -> TurnSlp/1
  Rim_turnv/1 -> Terminator6/1
  Sync_In/1 -> Terminator12/1
  Ground2/1 -> Alpha/1
  Ground3/1 -> LongFrc/1
  Ground4/1 -> SideFrc/1
  Ground5/1 -> OverturnTrq/1
  vxtrans/1 -> Terminator1/1
  vytrans/1 -> Terminator2/1
  Rim_rotv/1 -> Terminator3/1
  InclinAngle/1 -> Terminator4/1
  muRoad/1 -> Terminator5/1
  Load/1 -> Terminator/1
  Ground1/1 -> Slp/1
  Ground6/1 -> LoadFrc/1
  Ground7/1 -> RollResist/1
  Ground8/1 -> AlignTrq/1

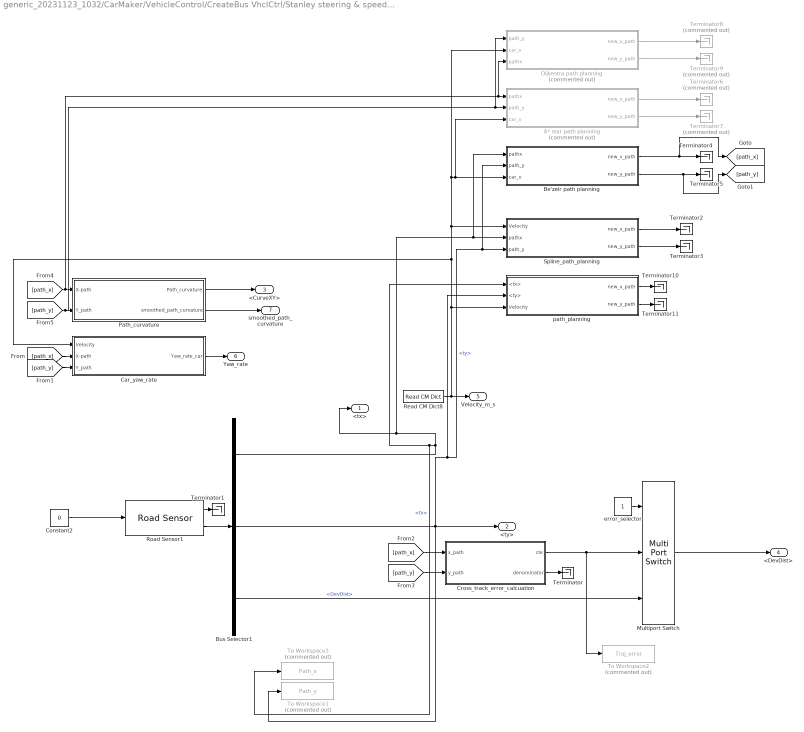
== system generic_20231123_1032/CarMaker/VehicleControl/CreateBus VhclCtrl/Stanley steering & speed//Brake controller/Road sensor set & path planning/Road sensor set & path planning ==
  A* star path planning : Subsystem  Commented=on
  Be'zeir path planning : Subsystem
  Bus Selector1 : BusSelector  OutputSignals=Path.tx,Path.ty,Path.DevDist
  Car_yaw_rate : Subsystem
  Constant2 : Constant  Value=0
  Cross_track_error_calcuation : Subsystem
  Dijkestra path planning : Subsystem  Commented=on
  Multiport Switch : MultiPortSwitch  Inputs=2  SaturateOnIntegerOverflow=off  InputSameDT=off
  Path_curvature : Subsystem
  Read CM Dict8 : CarMaker4SL/Read CM Dict  xname=Vhcl.v  xsync=off  xstime=Continuous
  Road Sensor1 : CarMaker4SL/Sensors/Road Sensor  xname=0  xstime=Continuous
      settings: SourceProductName=CarMaker4SL
  Spline_path_planning : Subsystem
  Terminator{,1..5,10..11} (8 alike) : Terminator
  Terminator{6..9} (4 alike) : Terminator  Commented=on
  To Workspace1 : ToWorkspace  Commented=on  VariableName=Path_y  SampleTime=-1
      settings: Save2DSignal=2-D array (concatenate along first dimension)
  To Workspace2 : ToWorkspace  Commented=on  VariableName=Traj_error  SampleTime=-1
      settings: Save2DSignal=2-D array (concatenate along first dimension)
  To Workspace3 : ToWorkspace  Commented=on  VariableName=Path_x  SampleTime=-1
      settings: Save2DSignal=2-D array (concatenate along first dimension)
  error_selector : Constant
  path_planning : Subsystem
  <tx> : Outport
  <ty> : Outport  Port=2
  <CurveXY> : Outport  Port=3
  <DevDist> : Outport  Port=4
  Velocity_m_s : Outport  Port=5
  Yaw_rate : Outport  Port=6
  smoothed_path_curvature : Outport  Port=7
  wires:
  [path_x] -> Car_yaw_rate/2(X-path)
  [path_x] -> Cross_track_error_calcuation/1(x_path)
  Bus Selector1/2 -> Be'zeir path planning/2(path_y), Spline_path_planning/3(path_y), path_planning/2(<ty>), To Workspace1/1, <ty>/1  "<ty>"
  Road Sensor1/2 -> Bus Selector1/1
  Constant2/1 -> Road Sensor1/1
  Path_curvature/1(Path_curvature) -> <CurveXY>/1
  Road Sensor1/1 -> Terminator1/1
  [path_y] -> Cross_track_error_calcuation/2(y_path)
  [path_y] -> Car_yaw_rate/3(Y_path)
  Bus Selector1/1 -> path_planning/1(<tx>), To Workspace3/1, Be'zeir path planning/1(pathx), Spline_path_planning/2(pathx), <tx>/1  "<tx>"
  Bus Selector1/3 -> Multiport Switch/3  "<DevDist>"
  error_selector/1 -> Multiport Switch/1
  Cross_track_error_calcuation/1(cte) -> To Workspace2/1, Multiport Switch/2
  Cross_track_error_calcuation/2(denominator) -> Terminator/1
  Car_yaw_rate/1(Yaw_rate_car) -> Yaw_rate/1
  path_planning/1(new_x_path) -> Terminator10/1
  path_planning/2(new_y_path) -> Terminator11/1
  Multiport Switch/1 -> <DevDist>/1
  Path_curvature/2(smoothed_path_curvature) -> smoothed_path_curvature/1
  Spline_path_planning/2(new_y_path) -> Terminator3/1
  Spline_path_planning/1(new_x_path) -> Terminator2/1
  Be'zeir path planning/1(new_x_path) -> [path_x], Terminator4/1
  Be'zeir path planning/2(new_y_path) -> [path_y], Terminator5/1
  [path_y] -> Dijkestra path planning/1(path_y), A* star path planning/2(path_y), Path_curvature/2(Y_path)
  [path_x] -> Dijkestra path planning/3(pathx), A* star path planning/1(pathx), Path_curvature/1(X-path)
  A* star path planning/2(new_y_path) -> Terminator7/1
  A* star path planning/1(new_x_path) -> Terminator6/1
  Dijkestra path planning/1(new_x_path) -> Terminator8/1
  Dijkestra path planning/2(new_y_path) -> Terminator9/1
  Read CM Dict8/1 -> Dijkestra path planning/2(car_v), A* star path planning/3(car_v), Be'zeir path planning/3(car_v), Spline_path_planning/1(Velocity), Car_yaw_rate/1(Velocity), path_planning/3(Velocity), Velocity_m_s/1

== system generic_20231123_1032/CarMaker/VehicleControl/CreateBus VhclCtrl/Stanley steering & speed//Brake controller/Stanley controller with path_planning/Stanley controller with path_planning ==
  X-path : Inport
  Y_path : Inport  Port=2
  Discrete-Time Integrator1 : DiscreteIntegrator  Commented=on  SampleTime=-1  ICPrevOutput=DiscIntNeverNeededParam  ICPrevScaledInput=DiscIntNeverNeededParam
  MATLAB Function : MATLAB Function  Commented=on  TreatAsAtomicUnit=on
  MATLAB Function1 : MATLAB Function  Commented=on  TreatAsAtomicUnit=on
  Path_Calculation_V02 : MATLAB Function  Commented=on  TreatAsAtomicUnit=on
  Read CM Dict10 : CarMaker4SL/Read CM Dict  Commented=on  xname=Vhcl.v  xsync=off  xstime=Continuous
  Read CM Dict11 : CarMaker4SL/Read CM Dict  Commented=on  xname=Car.Gen.tx  xsync=off  xstime=Continuous
  Read CM Dict13 : CarMaker4SL/Read CM Dict  Commented=on  xname=Car.YawRate  xsync=off  xstime=Continuous
  Read CM Dict7 : CarMaker4SL/Read CM Dict  Commented=on  xname=Car.Road.Path.DevDist  xsync=off  xstime=Continuous
  Read CM Dict9 : CarMaker4SL/Read CM Dict  Commented=on  xname=Car.Gen.ty  xsync=off  xstime=Continuous
  Saturation : Saturate  Commented=on  UpperLimit=1.6  LowerLimit=-1.6
  Subsystem3 : Subsystem  Commented=on
  X_Global_Pos_m : Subsystem  Commented=on
  Y_Global_Pos_m : Subsystem  Commented=on
  Yaw_angle_rad : Subsystem  Commented=on
  e : Outport
  err_fr_axle : Outport  Port=2
  cross_track_steering : Outport  Port=3
  heading_err : Outport  Port=4
  Steering : Outport  Port=5
  closest_point : Outport  Port=6
  wires:
  X-path/1 -> Subsystem3/1(X-path)
  MATLAB Function/5(steering) -> Saturation/1
  X_Global_Pos_m/1(Pos_X) -> MATLAB Function1/1(Pos_X)
  Y_path/1 -> Subsystem3/2(Y_path)
  Subsystem3/1(x_path) -> Path_Calculation_V02/3(path_x)
  Read CM Dict13/1 -> Discrete-Time Integrator1/1, MATLAB Function/3(yaw)
  Read CM Dict9/1 -> Y_Global_Pos_m/1(In1), Path_Calculation_V02/2(y_car)
  Read CM Dict11/1 -> X_Global_Pos_m/1(In1), Path_Calculation_V02/1(x_car)
  Subsystem3/2(y_path) -> Path_Calculation_V02/4(y_path)
  Discrete-Time Integrator1/1 -> Yaw_angle_rad/1(In1)
  Y_Global_Pos_m/1(Pos_Y) -> MATLAB Function1/2(Pos_Y)
  Path_Calculation_V02/1(closest_point) -> closest_point/1
  Path_Calculation_V02/2(instantaneous_path) -> MATLAB Function1/4(Path_In)
  Yaw_angle_rad/1(Yaw_Angle) -> MATLAB Function1/3(Yaw_Angle)
  MATLAB Function1/1(Path_Out) -> MATLAB Function/1(path)
  Read CM Dict7/1 -> MATLAB Function/2(dev)
  Read CM Dict10/1 -> MATLAB Function/4(speed_act)
  MATLAB Function/1(e) -> e/1
  MATLAB Function/2(err_fr_axle) -> err_fr_axle/1
  MATLAB Function/3(cross_track_steering) -> cross_track_steering/1
  MATLAB Function/4(heading_err) -> heading_err/1
  Saturation/1 -> Steering/1  "Steering"

== system generic_20231123_1032/CarMaker/VehicleControl/CreateBus VhclCtrl/Stanley steering & speed//Brake controller/Stanley_controller_vfin/Stanley_controller_vfin ==
  Velocity : Inport
  Curvature : Inport  Port=2
  Vehicle_yaw_rate : Inport  Port=3
  Path.DevDist : Inport  Port=4
  Stanley_standfort controller : Subsystem  VariantControl=Choice
  Steering angle : Outport
  dev_angle : Outport  Port=2

== system generic_20231123_1032/CarMaker/VehicleControl/CreateBus VhclCtrl/Stanley steering & speed//Brake controller/Stanley_controller_with_thottle_and_brake_commands/MPCLongitudianl_contorl ==
  smoothed_path_curvature : Inport
  Desired_speed : Inport  Port=2
  steering_angle : Inport  Port=3
  Abs : Abs  SaturateOnIntegerOverflow=off
  Compare To Constant : simulink/Logic and Bit Operations/Compare To Constant  relop=>=  const=0.5  OutDataTypeStr=boolean
  Compare To Constant1 : simulink/Logic and Bit Operations/Compare To Constant  relop=<  const=0.5  OutDataTypeStr=boolean
  Compare To Constant2 : simulink/Logic and Bit Operations/Compare To Constant  relop=<=  const=1.5  OutDataTypeStr=boolean
  Constant : Constant  Value=0
  Constant1 : Constant
  Constant3 : Constant  Value=A
  Constant4 : Constant  Value=B
  Gain : Gain  Gain=-1
  MATLAB Function1 : MATLAB Function  Commented=on  TreatAsAtomicUnit=on
  MPC_speed_control : MATLAB Function  TreatAsAtomicUnit=on
  NOT : Logic  Operator=NOT  IconShape=distinctive  AllPortsSameDT=off  OutDataTypeStr=boolean
  Product : Product
  Product1 : Product
  Read CM Dict : CarMaker4SL/Read CM Dict  xname=Vhcl.v  xsync=off  xstime=Continuous
  Speed_regulator : Subsystem
  Switch : Switch  Criteria=u2 > Threshold  SaturateOnIntegerOverflow=off  InputSameDT=off
  Switch1 : Switch  Criteria=u2 ~= 0  SaturateOnIntegerOverflow=off  InputSameDT=off
  actual_velocity : Outport
  Deisred_speed : Outport  Port=2
  throttle : Outport  Port=3
  Brake : Outport  Port=4
  wires:
  Read CM Dict/1 -> Speed_regulator/4(current_speed), actual_velocity/1, Speed_regulator/1(Actual_velocity)
  Abs/1 -> Gain/1
  Speed_regulator/2(desired_speed) -> Compare To Constant2/1, Deisred_speed/1
  steering_angle/1 -> Speed_regulator/5(steering_angle)
  Speed_regulator/1(speed_error) -> Compare To Constant1/1, Abs/1, Compare To Constant/1  "speed_error"
  Desired_speed/1 -> Speed_regulator/2(Desired_speed)
  smoothed_path_curvature/1 -> Speed_regulator/3(smoothed_path_curvature)
  Gain/1 -> MPC_speed_control/1(speed_error)  "error"
  Constant4/1 -> MPC_speed_control/3(B)
  Constant3/1 -> MPC_speed_control/2(A)
  Compare To Constant2/1 -> Switch1/2, NOT/1
  NOT/1 -> Switch/2
  Constant/1 -> Switch/3
  Compare To Constant1/1 -> Product/2
  Switch/1 -> Product1/1, Product/1
  Compare To Constant/1 -> Product1/2
  Product/1 -> throttle/1
  Constant1/1 -> Switch1/1
  Product1/1 -> Switch1/3
  Switch1/1 -> Brake/1
  MPC_speed_control/1(throttle_Brake) -> Switch/1

== system generic_20231123_1032/CarMaker/VehicleControl/CreateBus VhclCtrl/Stanley steering & speed//Brake controller/Stanley_controller_with_thottle_and_brake_commands/Stanley steering + PID speed controller ==
  Path_out : Inport
  <Vx_Global_m_s> : Inport  Port=2
  <Vy_Global_m_s> : Inport  Port=3
  dev_angle : Inport  Port=4
  <Actual_Velocity_Car_m_s> : Inport  Port=5
  Desired_speed : Inport  Port=6
  dev_distance : Inport  Port=7
  Actual velocity [km/h] : Display
  Bus Selector : BusSelector  OutputSignals=Path.tx,Path.ty
  Constant1 : Constant  Value=0
  Delay : Delay  DelayLength=1
  Delay1 : Delay  DelayLength=1
  Gain : Gain  Gain=3.6
  Road Sensor : CarMaker4SL/Sensors/Road Sensor  xname=0  xstime=Continuous
      settings: SourceProductName=CarMaker4SL
  Saturation : Saturate  UpperLimit=pi()/2  LowerLimit=-pi/2
  Smoothing : Subsystem
  Speed_controller : Subsystem
  Stanely_controller : MATLAB Function  TreatAsAtomicUnit=on
  Subsystem1 : Subsystem
  Terminator : Terminator
  Terminator1 : Terminator
  Terminator4 : Terminator
  Steering_angle_rad : Outport  VectorParamsAs1DForOutWhenUnconnected=off
  Throttle : Outport  Port=2
  Brake_command : Outport  Port=3
  wires:
  dev_distance/1 -> Stanely_controller/2(dev)  "Dev_dis[m]"
  <Vx_Global_m_s>/1 -> Speed_controller/3(velocity_x)
  Constant1/1 -> Road Sensor/1
  dev_angle/1 -> Stanely_controller/1(dev_angle)  "dev_angle [rad]"
  <Vy_Global_m_s>/1 -> Speed_controller/4(velocity_y)
  Bus Selector/2 -> Stanely_controller/6(y2), Delay1/1  "<ty>"
  Speed_controller/4(min_safe_speed) -> Subsystem1/3(min_safe_speed)
  Road Sensor/1 -> Terminator4/1
  Road Sensor/2 -> Bus Selector/1
  Bus Selector/1 -> Stanely_controller/4(x2), Delay/1  "<tx>"
  Delay/1 -> Stanely_controller/3(x1)
  Delay1/1 -> Stanely_controller/5(y1)
  <Actual_Velocity_Car_m_s>/1 -> Speed_controller/2(speed_act), Gain/1, Stanely_controller/7(speed_act)
  Desired_speed/1 -> Subsystem1/1(desired_speed)
  Speed_controller/2(Brake_command) -> Brake_command/1
  Stanely_controller/3(steering) -> Speed_controller/6(steering), Saturation/1  "steering"
  Gain/1 -> Actual velocity [km/h]/1  "Actual velocity [km/h]"
  Path_out/1 -> Speed_controller/1(path)
  Subsystem1/1(Target_speed) -> Speed_controller/5(desired_speed)
  Saturation/1 -> Smoothing/1(Signal_In)  "Control signal"
  Speed_controller/1(Throttle) -> Throttle/1
  Speed_controller/3(path_curvature) -> Subsystem1/2(curvature)
  Smoothing/1(Signal_Out) -> Steering_angle_rad/1
  Stanely_controller/2(cross_track_steering) -> Terminator/1  "cross_track_steering"
  Stanely_controller/1(e) -> Terminator1/1  "cross track error [m]"

== system generic_20231123_1032/CarMaker/VehicleControl/CreateBus VhclCtrl/Stanley steering & speed//Brake controller/Road sensor set & path planning/Road sensor set & path planning/A* star path planning ==
  pathx : Inport
  path_y : Inport  Port=2
  car_v : Inport  Port=3
  Basic_obstacle avoidance : MATLAB Function  TreatAsAtomicUnit=on
  Demux : Demux  Commented=on
  Discrete-Time Integrator : DiscreteIntegrator  SampleTime=-1  ICPrevOutput=DiscIntNeverNeededParam  ICPrevScaledInput=DiscIntNeverNeededParam
  Display : Display
  Mux : Mux  Inputs=2
  Mux1 : Mux  Inputs=2
  Read CM Dict : CarMaker4SL/Read CM Dict  xname=Sensor.Object.RadarL.Obj.T00.RefPnt.ds.x  xsync=off  xstime=Continuous
  Read CM Dict1 : CarMaker4SL/Read CM Dict  xname=Sensor.Object.RadarL.Obj.T00.RefPnt.ds.y  xsync=off  xstime=Continuous
  Read CM Dict2 : CarMaker4SL/Read CM Dict  xname=Car.Gen.tx  xsync=off  xstime=Continuous
  Read CM Dict3 : CarMaker4SL/Read CM Dict  xname=Car.Gen.ty  xsync=off  xstime=Continuous
  Read CM Dict4 : CarMaker4SL/Read CM Dict  xname=Sensor.Radar.VehSensor_6.Obj0.Width  xsync=off  xstime=Continuous
  Read CM Dict5 : CarMaker4SL/Read CM Dict  xname=Sensor.Radar.VehSensor_6.Obj0.Length  xsync=off  xstime=Continuous
  Read CM Dict6 : CarMaker4SL/Read CM Dict  xname=Car.YawRate  xsync=off  xstime=Continuous
  Reshape : Reshape  OutputDimensionality=Customize  OutputDimensions=[2,1]
  Reshape1 : Reshape  OutputDimensionality=Customize  OutputDimensions=[1,2]
  Reshape4 : Reshape  Commented=on
  Saturation : Saturate  UpperLimit=4  LowerLimit=-4
  Signal_smoothing : Subsystem
  Smoothing3 : Subsystem
  getInstantaneousPath Function : MATLAB Function  Commented=on  TreatAsAtomicUnit=on
  lookahead_dist : Constant  Commented=on  Value=2
  new_x_path : Outport
  new_y_path : Outport  Port=2
  wires:
  Reshape4/1 -> Demux/1
  Demux/4 -> new_y_path/1
  Basic_obstacle avoidance/1(updated_path) -> getInstantaneousPath Function/1(generated_path), Display/1, Reshape4/1
  Demux/1 -> new_x_path/1
  lookahead_dist/1 -> getInstantaneousPath Function/2(lookahead_distance)
  pathx/1 -> Basic_obstacle avoidance/8(path_x), Mux1/1
  path_y/1 -> Basic_obstacle avoidance/9(path_y), Mux1/2
  car_v/1 -> Basic_obstacle avoidance/7(car_v)
  Smoothing3/1(Signal_Out) -> Basic_obstacle avoidance/5(object_length)  "steering_signal"
  Signal_smoothing/1(smoothed_width) -> Basic_obstacle avoidance/6(object_width)
  Saturation/1 -> Smoothing3/1(Signal_In)
  Discrete-Time Integrator/1 -> getInstantaneousPath Function/4(current_heading)
  Reshape/1 -> getInstantaneousPath Function/3(current_position)
  Mux1/1 -> Reshape1/1
  Read CM Dict5/1 -> Saturation/1
  Read CM Dict6/1 -> Discrete-Time Integrator/1
  Mux/1 -> Reshape/1
  Read CM Dict3/1 -> Basic_obstacle avoidance/2(Car_y), Mux/2
  Read CM Dict4/1 -> Signal_smoothing/1(Signal_In)
  Read CM Dict2/1 -> Basic_obstacle avoidance/1(Car_x), Mux/1
  Read CM Dict1/1 -> Basic_obstacle avoidance/4(dy)
  Read CM Dict/1 -> Basic_obstacle avoidance/3(dx)
